simulink model "Pract6_3PID2Salidas"  (R2012b)
settings: Solver=ode45  StartTime=0.0  StopTime=10  RelTol=1e-3
PreLoadFcn:
  | M = 0.5;
  | m = 0.2;
  | b = 0.1;
  | I = 0.006;
  | g = 9.8;
  | l = 0.3;
  | q = (M+m)*(I+m*l^2)-(m*l)^2;
libraries: simulink x1
settings Model: Creator=Aitor  LastModifiedBy=Aitor

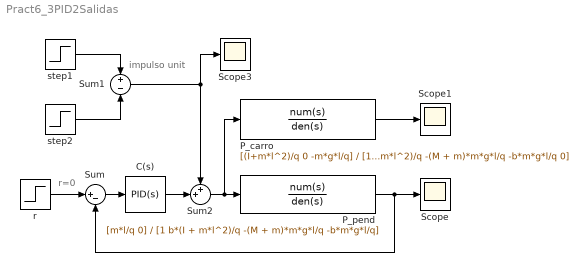
== system Pract6_3PID2Salidas ==
  note: r=0
  note: impulso unit
  C(s) : simulink/Continuous/PID Controller  Controller=PID  TimeDomain=Continuous-time  SampleTime=1  IntegratorMethod=Forward Euler  FilterMethod=Forward Euler  Form=Parallel  P=100  I=100  D=50  N=1000  InitialConditionSource=internal  InitialConditionForIntegrator=0  InitialConditionForFilter=0  ExternalReset=none  LimitOutput=off  UpperSaturationLimit=inf  LowerSaturationLimit=-inf  LinearizeAsGain=on  AntiWindupMode=none  Kb=1  TrackingMode=off  Kt=1  PParamMin=[]  PParamMax=[]  IParamMin=[]  IParamMax=[]  DParamMin=[]  DParamMax=[]  NParamMin=[]  NParamMax=[]  KbParamMin=[]  KbParamMax=[]  KtParamMin=[]  KtParamMax=[]  POutMin=[]  POutMax=[]  IOutMin=[]  IOutMax=[]  DOutMin=[]  DOutMax=[]  NOutMin=[]  NOutMax=[]  KbOutMin=[]  KbOutMax=[]  KtOutMin=[]  KtOutMax=[]  IntegratorOutMin=[]  IntegratorOutMax=[]  FilterOutMin=[]  FilterOutMax=[]  SumOutMin=[]  SumOutMax=[]  SumI1OutMin=[]  SumI1OutMax=[]  SumI2OutMin=[]  SumI2OutMax=[]  SumI3OutMin=[]  SumI3OutMax=[]  SumDOutMin=[]  SumDOutMax=[]  SaturationOutMin=[]  SaturationOutMax=[]  IntegratorContinuousStateAttributes=''  IntegratorStateMustResolveToSignalObject=off  IntegratorRTWStateStorageClass=Auto  FilterContinuousStateAttributes=''  FilterStateMustResolveToSignalObject=off  FilterRTWStateStorageClass=Auto
  P_carro : TransferFcn  Numerator=[(I+m*l^2)/q 0 -m*g*l/q]  Denominator=[1 b*(I + m*l^2)/q -(M + m)*m*g*l/q -b*m*g*l/q 0]
  "P_pend " : TransferFcn  Numerator=[m*l/q 0]  Denominator=[1 b*(I + m*l^2)/q -(M + m)*m*g*l/q -b*m*g*l/q]
  Scope : Scope
      settings: YMin=-0.2  YMax=0.2
  Scope1 : Scope
      settings: YMin=-5.05e+09  YMax=-4.3e+09
  Scope3 : Scope
      settings: YMin=0  YMax=1.4  SaveName=ScopeData3
  Sum : Sum  Inputs=|+-
  Sum1 : Sum  Inputs=+|-
  Sum2 : Sum  Inputs=++|
  r : Step  Time=0  After=0  SampleTime=0
  step1 : Step  Time=0  After=1e6  SampleTime=0
  step2 : Step  Time=1/1e6  After=1e6  SampleTime=0
  wires:
  r/1 -> Sum/1
  Sum/1 -> C(s)/1
  "P_pend "/1 -> Scope/1, Sum/2
  step1/1 -> Sum1/1
  step2/1 -> Sum1/2
  C(s)/1 -> Sum2/2
  Sum2/1 -> P_carro/1, "P_pend "/1
  Sum1/1 -> Sum2/1, Scope3/1
  P_carro/1 -> Scope1/1
